simulink model "mcc_audio"  (R2012b)
settings: Solver=FixedStepDiscrete  StartTime=0.0  StopTime=10  FixedStep=0.01  RelTol=1e-3
undefined symbols (not defined in the file or in its folder): analoginput, analogoutput
libraries: daqlib x2
settings Model: Creator=armigrs1  LastModifiedBy=armigrs1

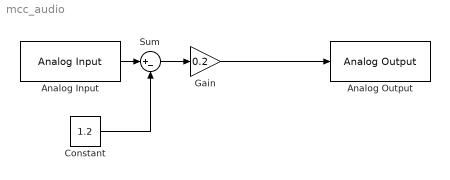
== system mcc_audio ==
  Analog Input : daqlib/Analog Input  AcqMode=0  DeviceMenu=mcc 0 (USB-1208FS)  Device=mcc 0 (USB-1208FS)  ObjConstructor=analoginput('mcc',0)  SampleRate=5000  ActualRate=5000  SamplesPerFrame=2000  InputType=SingleEnded  NChannelsSelected=2  Channels=1$0$$1$#1$1$$1$#0$2$$1$#0$3$$1$#0$4$$1$#0$5$$1$#0$6$$1$#0$7$$1$#  NPorts=1 for all hardware channels  DataType=double
      settings: SignalType=Sample-based
  Analog Output : daqlib/Analog Output  OutMode=0  DeviceMenu=winsound 0 (Microphone Array (IDT High Defi)  Device=winsound 0 (Microphone Array (IDT High Defi)  ObjConstructor=analogoutput('winsound',0)  OutputRate=5000  ActualRate=5000  NChannelsSelected=2  Channels=1$1$Left$1$N/A$#1$2$Right$1$N/A$#  NPorts=1 for all hardware channels
  Constant : Constant  Value=1.2
  Gain : Gain  Gain=0.2
  Sum : Sum  Inputs=|+-
  wires:
  Gain/1 -> Analog Output/1
  Analog Input/1 -> Sum/1
  Sum/1 -> Gain/1
  Constant/1 -> Sum/2
